simulink model "Aenea_model"  (R2020b)
settings: Solver=FixedStepDiscrete  StartTime=0.0  StopTime=10.0  FixedStep=0.02  RelTol=1e-3
values from neighbouring files (symbols this model uses):
  attuatore_Amax = deg2rad(27)    [AVVIO_AENEA_DATA.m]
  attuatore_Amin = deg2rad(-23)    [AVVIO_AENEA_DATA.m]
  attuatore_Emax = deg2rad(18)    [AVVIO_AENEA_DATA.m]
  attuatore_Emin = deg2rad(-32)    [AVVIO_AENEA_DATA.m]
  attuatore_Rmax = deg2rad(30)    [AVVIO_AENEA_DATA.m]
  attuatore_Rmin = deg2rad(-30)    [AVVIO_AENEA_DATA.m]
  attuatore_Tmax = 1    [AVVIO_AENEA_DATA.m]
  attuatore_Tmin = 0    [AVVIO_AENEA_DATA.m]
  interventoA_05 = 25    [AVVIO_AENEA_DATA.m]
  interventoA_1 = 20    [AVVIO_AENEA_DATA.m]
  interventoE_05 = 20    [AVVIO_AENEA_DATA.m]
  interventoE_1 = 15    [AVVIO_AENEA_DATA.m]
  interventoT = 0.1    [AVVIO_AENEA_DATA.m]
  inv_A = -1    [AVVIO_AENEA_DATA.m]
  inv_comp_h = -1    [AVVIO_AENEA_DATA.m]
  inv_E = 1    [AVVIO_AENEA_DATA.m]
  inv_R = 1    [AVVIO_AENEA_DATA.m]
  inv_T = 1    [AVVIO_AENEA_DATA.m]
  K_AW_B_AP_quota = 1000    [AVVIO_AENEA_DATA.m]
  K_AW_B_becc = -250    [AVVIO_AENEA_DATA.m]
  K_AW_B_imb = 0    [AVVIO_AENEA_DATA.m]
  K_AW_B_roll = 500    [AVVIO_AENEA_DATA.m]
  K_imb_inv = -1    [AVVIO_AENEA_DATA.m]
  Kd_h_app = 0.085    [AVVIO_AENEA_DATA.m]
  Kd_h_flare = 0.01    [AVVIO_AENEA_DATA.m]
  Ki_AP_quota_select = 0.014    [AVVIO_AENEA_DATA.m]
  Ki_AP_rotta = 0.03    [AVVIO_AENEA_DATA.m]
  Ki_AP_vel = 0.001*8    (= 0.008)    [AVVIO_AENEA_DATA.m]
  Ki_becch = -0.064065*10    (= -0.64065)    [AVVIO_AENEA_DATA.m]
  Ki_h_app = 0.055    [AVVIO_AENEA_DATA.m]
  Ki_h_cruise = 0.008    [AVVIO_AENEA_DATA.m]
  Ki_h_flare = 0.07    [AVVIO_AENEA_DATA.m]
  Ki_roll = 0.025*10    (= 0.25)    [AVVIO_AENEA_DATA.m]
  Kp_AP_quota_hold_h = 0.15    [AVVIO_AENEA_DATA.m]
  Kp_AP_quota_hold_l = 1    [AVVIO_AENEA_DATA.m]
  Kp_AP_quota_select = 0.014    [AVVIO_AENEA_DATA.m]
  Kp_AP_rotta = 0.7    [AVVIO_AENEA_DATA.m]
  Kp_AP_vel = 0.2692/8    (= 0.03365)    [AVVIO_AENEA_DATA.m]
  Kp_becch = -0.1918*10    (= -1.918)    [AVVIO_AENEA_DATA.m]
  Kp_comp_h = 0.035*15    (= 0.525)    [AVVIO_AENEA_DATA.m]
  Kp_h_app_max = 0.086    [AVVIO_AENEA_DATA.m]
  Kp_h_app_min = 0.01    [AVVIO_AENEA_DATA.m]
  Kp_h_cruise = 0.04    [AVVIO_AENEA_DATA.m]
  Kp_h_flare = 0.1    [AVVIO_AENEA_DATA.m]
  Kp_imb = -0.04*10    (= -0.4)    [AVVIO_AENEA_DATA.m]
  Kp_p = 0.025*5    (= 0.125)    [AVVIO_AENEA_DATA.m]
  Kp_q = -0.025*5    (= -0.125)    [AVVIO_AENEA_DATA.m]
  Kp_roll = 0.11*10    (= 1.1)    [AVVIO_AENEA_DATA.m]
  Kp_Rotta_ATO = 4    [AVVIO_AENEA_DATA.m]
  phi_max = deg2rad(30)    [AVVIO_AENEA_DATA.m]
  phi_min = deg2rad(-30)    [AVVIO_AENEA_DATA.m]
  pwm_aileron_max = 1940    [AVVIO_AENEA_DATA.m]
  pwm_aileron_min = 1099    [AVVIO_AENEA_DATA.m]
  pwm_elevator_max = 1939    [AVVIO_AENEA_DATA.m]
  pwm_elevator_min = 1099    [AVVIO_AENEA_DATA.m]
  pwm_rudder_max = 1971    [AVVIO_AENEA_DATA.m]
  pwm_rudder_min = 1130    [AVVIO_AENEA_DATA.m]
  pwm_throttle_max = 1940    [AVVIO_AENEA_DATA.m]
  pwm_throttle_min = 1160    [AVVIO_AENEA_DATA.m]
  safe_phi = 55    [AVVIO_AENEA_DATA.m]
  safe_V = 40    [AVVIO_AENEA_DATA.m]
  t_AP = 0.02    [AVVIO_AENEA_DATA.m]
  theta_max = deg2rad(15)    [AVVIO_AENEA_DATA.m]
  theta_min = deg2rad(-15)    [AVVIO_AENEA_DATA.m]
  time_alarm_SAFE = 1    [AVVIO_AENEA_DATA.m]
  V_max = 30    [AVVIO_AENEA_DATA.m]
  V_stall = 11    [AVVIO_AENEA_DATA.m]
  vel_wp1_al = 25    [AVVIO_AENEA_DATA.m]
  vel_wp2_al = 20    [AVVIO_AENEA_DATA.m]
undefined symbols (not defined in the file or in its folder): bias, DiscIntNeverNeededParam, Newton, Q1B, R1B, Raphson, Sensor_Offsets, tsamp, UP, vd_ini
libraries: simulink_extras x41, slpidlib x8, simulink x6, dspsigops x4, arduinolib x3, svdutilitieslib x3, aerolibtransform2sys x2, aerolibtransform2 x2, aerosimlib x2, cstblocks x1
(part 7 of 8)

== matlab function Aenea_model/AUTOPILOT_MODEL/AIR RX/MATLAB Function4 ==
  data: byte_pack input; status output; messaggio output; messaggio_2 output; byte_available input
function [status,messaggio,messaggio_2]  = Creazione_mavlink_message_2(byte_pack,byte_available)


persistent Interr_parz  message counter len_found mess_len

if isempty(Interr_parz)
    Interr_parz = false ;
end
if isempty(message)
     message = uint8(zeros(1,100 )) ;
end
if isempty (counter) 
    counter = uint8(0) ;    % variabile che conta quanti byte mancano per completare il messaggio
end 

if isempty(len_found) 
     len_found = false ;
end 

if isempty(mess_len) 
     mess_len = 0 ;
end 

status = 0;
M = length(byte_pack) ;
caso = 0 ;
messaggio = uint8(zeros(1,100 )) ;
messaggio_2 = uint8(zeros(1,100 )) ;
% LA VARIABILE INTERR_PARZ va attivata a 1 alla fine della funzone di
% lettura per indicare di leggere il successivo messaggio in arrivo 

[poss_254,num_254] = find_254(byte_pack) ;

if ((Interr_parz == true) && (num_254 == 1))                  % in questo caso verifico che il 254 sia effettivamente un altro inizio
if (poss_254(1) ~= counter+1)
   num_254 = 0; 
end
    
end



if ( num_254 == 1 && Interr_parz == false )             
    caso = 1 ;                                                            % 1 Messaggio Intero   o parziale che inizia                % attivare alla fine della funzione Interr_parz == true o false 
elseif (num_254 == 0 && Interr_parz == true )
    caso = 2 ;                                                        % 1 Messaggio Parziale senza inizio e poi nulla 
elseif (num_254 == 1 && Interr_parz == true )                         
    caso = 3 ;                                                        % 1 Messaggio Parziale e poi un altro messaggio completo o parziale
elseif  ( num_254 == 2 && Interr_parz == false ) 
    caso = 4 ;                                                         % Due messaggi completi  oppure 1 Completo + parziale ( attivare Interr_parz alla fine del codice)
end


switch (caso)
   
    
    
    case 1 
        pos_254 = poss_254(num_254) ;
        
        if pos_254 == M                                                                          % se il 254 sta alla fine 
             message(1) = byte_pack(pos_254)  ;
            len_found = false ;
            Interr_parz = true ;
        else
             len = byte_pack(pos_254 + 1)  ;
             if len <= 100
             if  ((byte_pack(poss_254(1)+1) + 8) == byte_available)                                             % se abbiamo tutto il messaggio all'interno del byte_pack
                message(1: 8 + len ) = byte_pack(pos_254 : pos_254 + (7+len) ) ;          % era cosi byte_pack(pos_254 : pos_254 + (8+len) ) ;
                messaggio = message ;
                status = 1 ;
                message = uint8(zeros(1,100 )) ;
                counter = uint8(0) ;
                len_found = true ;
                mess_len = 0 ;
             elseif ((byte_pack(poss_254(1)+1) + 8) > byte_available)
                mess_len = double(byte_available) ;                                       % lunghezza del messaggio da leggere dal byte_pack ( non uguale alla lunghezza del messaggio complessivo)
                message(1 : mess_len) = byte_pack(pos_254 : mess_len ) ;
                len_found = true ;
                counter = 8 + len - mess_len ;
                Interr_parz = true ;
             end
             else
                 messaggio = uint8(zeros(1,100 )) ;              
                 Interr_parz = false;
                 message = uint8(zeros(1,100 )) ;
                 counter = uint8(0) ;
                 len_found = false ;
                 mess_len = 0 ; 
                 status = 1 ;
             end   
             
        end
        
        
        
        
    case 2 
        
                                     % se la lunghezza è stata trovata e quindi ho il valore di counter che indica quante componenti mancano
           if byte_pack ~= 0
                message(mess_len + 1 : mess_len + counter) = byte_pack( 1 : counter) ;
                Interr_parz = false ;
                messaggio = message ;
                status = 1 ;
                message = uint8(zeros(1,100 )) ;
                len_found = true ;
                mess_len = 0 ;
                counter = uint8(0) ;
                
           else                                                    % se ho un messaggio parziale e nello step successivo non ricevo nulla allora azzero tutto, altrimenti entro in un loop infinito di messaggi sbagliati
                Interr_parz = false ;
                messaggio = uint8(zeros(1,100)) ;
                status = 1 ;
                message = uint8(zeros(1,100 )) ;
                len_found = true ;
                mess_len = 0 ;
                counter = uint8(0) ;  
           end        
        
        

  
        
    case 3 
        
                                     % se la lunghezza è stata trovata e quindi ho il valore di counter che indica quante componenti mancano
        pos_254 = poss_254(num_254) ;
        
                message(mess_len + 1 : mess_len + counter) = byte_pack( 1 : counter) ;
                Interr_parz = false ;
                messaggio = message ;
                status = 1 ;
                message = uint8(zeros(1,100 )) ;
                len_found = true ;
                mess_len = 0 ;
                counter = uint8(0) ;
                
             len = byte_pack(pos_254 + 1)  ;
             if len <= 100
             if  ((byte_pack(poss_254(1)+1) + 8) == uint8(byte_available-double(counter)))                                             % se abbiamo tutto il messaggio all'interno del byte_pack
                message(1: 8 + len ) = byte_pack(pos_254 : pos_254 + (7+len) ) ;          % era cosi byte_pack(pos_254 : pos_254 + (8+len) ) ;
                messaggio_2 = message ;
                status = 1 ;
                message = uint8(zeros(1,100 )) ;
                counter = uint8(0) ;
                len_found = true ;
                mess_len = 0 ;
             elseif ((byte_pack(poss_254(1)+1) + 8) > (uint8(byte_available)-counter))
                mess_len = double(byte_available) - double(counter) ;                                       % lunghezza del messaggio da leggere dal byte_pack ( non uguale alla lunghezza del messaggio complessivo)
                message(1 : mess_len) = byte_pack(pos_254 : mess_len ) ;
                len_found = true ;
                counter = 8 + len - mess_len ;
                Interr_parz = true ;
             end
             else
                 messaggio = uint8(zeros(1,100 )) ;              
                 Interr_parz = false;
                 message = uint8(zeros(1,100 )) ;
                 counter = uint8(0) ;
                 len_found = false ;
                 mess_len = 0 ; 
                 status = 1 ;
             end
                
      
            
        
        
        
      
        
        
    case 4
        primo_254 = poss_254(1) ;
        secondo_254 = poss_254(2) ;
        len_primo = byte_pack(primo_254 + 1) ;
    %    messaggio(1 : len_primo + 8) = byte_pack(primo_254 : primo_254 + (len_primo + 7)) ;           %era cosi      byte_pack(primo_254 : secondo_254 - 1)  ;

        if len_primo <= 100
        messaggio(1 : len_primo + 8) = byte_pack(primo_254 : primo_254 + (len_primo + 7)) ;             %era cosi      byte_pack(primo_254 : secondo_254 - 1)  ;
        else
        messaggio = uint8(zeros(1,100 )) ;
        Interr_parz = false;
        message = uint8(zeros(1,100 )) ;
        counter = uint8(0) ;
        len_found = false ;
        mess_len = 0 ;
        end
        
        status = 1;
        
             len = byte_pack(secondo_254 + 1)  ;
             if (len <= 100 && (secondo_254-primo_254 > 3))
             if ( (byte_available - ( secondo_254))  == 7 + len    )                                         % se abbiamo tutto il messaggio all'interno del byte_pack
                message(1: 8 + len ) = byte_pack(secondo_254 : secondo_254 + (7+len) ) ;      % era cosi byte_pack(pos_254 : pos_254 + (8+len) ) ;
                messaggio_2 = message ;
                status = 2 ;
                message = uint8(zeros(1,100 )) ;
                counter = uint8(0) ;
                len_found = true ;
                mess_len = 0 ;
             else
                mess_len = length(byte_pack(secondo_254:byte_available ) ) ;    % lunghezza del messaggio da leggere dal byte_pack ( non uguale alla lunghezza del messaggio complessivo)
                message(1 : mess_len) = byte_pack(secondo_254:byte_available ) ;
                len_found = true ;
                counter = 8 + len - mess_len ;
                Interr_parz = true ;
             end
             else
               messaggio_2 = uint8(zeros(1,100 )) ;              
               Interr_parz = false;
               message = uint8(zeros(1,100 )) ;
               counter = uint8(0) ;
               len_found = false ;
               mess_len = 0 ;    
              end
             
        
        
end
end






function [position,counter] = find_254(pack) 
    position = zeros(1,3) ;
    
    M = length(pack)  ;   
    counter = 0 ;
    for i = 1 : M
        if pack(i) == 254 
            counter = counter + 1;  
            position(counter) = i; 
        end
    end
    l = pack(position(1)+1);
    if counter > 1
    if ((pack(l+8+position(1)) ~= 254) && (position(1) ~= 0))
        counter = 1;
        position(2) = 0;
    end
    end
end

== stateflow chart Aenea_model/AUTOPILOT_MODEL/AUTOPILOTA/Subsystem1/Chart ==
  state AutoTakeoff
    Wp_selector = 0;
    Vec_selector = 0;
    Ato_selector = 1;
    Al_selector = 0;
    Go_home_selector = 0;
  state Waypoint
    Wp_selector = 1;
    Vec_selector = 0;
    Ato_selector = 0;
    Al_selector = 0;
    Go_home_selector = 0;
  state In
    Wp_selector = 0;
    Vec_selector = 0;
    Ato_selector = 0;
    Al_selector = 0;
    Go_home_selector = 0;
  state AutoLanding
    Wp_selector = 0;
    Vec_selector = 0;
    Ato_selector = 0;
    Al_selector = 1;
    Go_home_selector = 0;
  state Vettoriale
    Wp_selector = 0;
    Vec_selector = 1;
    Ato_selector = 0;
    Al_selector = 0;
    Go_home_selector = 0;
  state GoHome
    Wp_selector = 0;
    Vec_selector = 0;
    Ato_selector = 0;
    Al_selector = 0;
    Go_home_selector = 1;
  AutoTakeoff -> Waypoint [order 2] : [Ap_sel == 1 && modo == 1]
  Waypoint -> In [order 2] : [Ap_sel == 0]
  AutoTakeoff -> In [order 1] : [Ap_sel == 0]
  (default) -> In : {Wp_selector = 0;
      | Vec_selector = 0;
      | Ato_selector = 0;
      | Al_selector = 0;}
  Waypoint -> AutoLanding [order 4] : [Ap_sel == 1 && modo == 4]
  In -> Waypoint [order 1] : [Ap_sel == 1 && modo == 1]
  In -> AutoTakeoff [order 5] : [Ap_sel == 1 && modo == 3]
  AutoLanding -> Waypoint [order 3] : [Ap_sel == 1 && modo == 1]
  AutoLanding -> In [order 1] : [Ap_sel == 0]
  Vettoriale -> In [order 1] : [Ap_sel == 0]
  AutoTakeoff -> Vettoriale [order 3] : [Ap_sel == 1 && modo == 2]
  Waypoint -> GoHome [order 1] : [Ap_sel == 1&& modo == 5]
  Waypoint -> Vettoriale [order 3] : [Ap_sel == 1 && modo == 2]
  Vettoriale -> Waypoint [order 2] : [Ap_sel == 1 && modo == 1]
  In -> AutoLanding [order 4] : [Ap_sel == 1 && modo == 4]
  In -> GoHome [order 3] : [Ap_sel == 1 && modo == 5]
  GoHome -> In : [Ap_sel == 0]
  In -> Vettoriale [order 2] : [Ap_sel == 1 && modo == 2]
  Vettoriale -> AutoLanding [order 4] : [Ap_sel == 1 && modo == 4]
  AutoLanding -> Vettoriale [order 2] : [Ap_sel == 1 && modo == 2]
  AutoLanding -> GoHome [order 4] : [Ap_sel == 1 && modo == 5]
  Vettoriale -> GoHome [order 3] : [Ap_sel == 1&& modo == 5]
  data: Al_selector output; Ato_selector output; Go_home_selector output; Vec_selector output; Wp_selector output; modo input; Ap_sel input

== stateflow chart Aenea_model/AUTOPILOT_MODEL/AIR TX/Enable /Chart ==
  state sendbyte(bt,n) [function]
  state Inputblock
    entry: i=1;
    Inputblock -> (junction 28)
    (junction 32) -> (junction 28) [order 1] : [ i<Len]
        | {i++;}
    (junction 28) -> (junction 32) : {sendbyte(datain,i);}
    (junction 32) -> (junction 48) [order 2] : {i=1;}
  (default) -> Inputblock
  data: bt function_input uint8; n function_input; datain input uint8; Len input uint16 size=1; i local uint8 =0

== stateflow chart Aenea_model/AUTOPILOT_MODEL/AUTOPILOTA/AUTOPILOTI1/CONTROLLORE DI QUOTA/SELEZIONE MODALITA' HOLD//SELECT ==
  state Select
    during:
    mod=1;
  state Hold
    during:
    mod=0;
  (default) -> Select
  Select -> Hold : [deltah<10]
  Hold -> Select : [deltah>10]
  data: mod output double; deltah input

== matlab function Aenea_model/AUTOPILOT_MODEL/AIR TX/Heartbeat/Alarm set ==
  data: Alarm input; H_mav output; Rx_mode input

%%

function H_mav = Allarm_set(Alarm, Rx_mode)
%#cambia lo stato se c'è un allarme attivo
% Allarm: possibili allarmi proveniente dall'autopilota
% Rx_mode: richiesta da parte della stazione di terra
% H_mav: setto i parametri Base_mode e System_status del Heartbeat


H_mav = uint8(Rx_mode); % setta la modalità con quella ricevuta da terra

% se un allarme si attiva ha la precedenza sulla richiesta della QGC

if Alarm(1) == 1 % ovvero l'aereo è entrato in safe e si pone su traettoria circolare di sicurezza
    
    H_mav(1) = uint8(220); % MAV_MODE_AUTO_ARMED
    H_mav(2) = uint8(5);   % MAV_STATE_CRITICAL
%     H_mav(3) = uint8(128); % MAV_MODE_FLAG_SAFETY_ARMED

end

% se l'allareme di intervento pilota è attivo ha precedenza sull'allarm
% sefe per cui bisogna riscrivere lo stato del pilota

if Alarm(2) == 1 % si è attivato l'allarme dell'intervento pilota 
    
    H_mav(1) = uint8(216); % MAV_MODE_GUIDED_ARMED
    H_mav(2) = uint8(4);   % MAV_STATE_ACTIVE
%     H_mav(3) = uint8(8);   % MAV_MODE_FLAG_GUIDED_ENABLED

end

== matlab function Aenea_model/AUTOPILOT_MODEL/AIR TX/If_subsystem/iflogic_function ==
  data: H50 input; iflogic output; H10 input
function iflogic = fcn(H50,H10)
%#codegen
% prende in ingeresso i counter che contano il tempo
% e dice quale messaggio bisogna inviare in base alle frequenze scelte in
% Heartbeat:            1Hz
% SCALED_IMU:           20Hz
%attitude:              20Hz
%GLOBAL_POSITION_INT:   1Hz
%SYS_STATUS:            3Hz
%VFR_HUD:               2Hz
%SERVO_OUTPUT_RAW       1Hz
%SCALED_PRESSURE        1Hz

if H50 == 1  || H50==3
    iflogic=uint8(26); % SCALED_IMU 20Hz
elseif H50==2 || H50==4
    iflogic=uint8(30); %attitude 20Hz
elseif  H50==0 && H10==2
    iflogic=uint8(33); %GLOBAL_POSITION_INT 1Hz
elseif  H50==0 && H10==6
    iflogic=uint8(34); %GLOBAL_POSITION_INT_RAW 1Hz
elseif  H50==0 && H10==0
    iflogic=uint8(0); %Heartbeat 1Hz
elseif H50==0 && (H10==1 || H10==5 || H10==9)
    iflogic=uint8(1); %SYS_STATUS 3Hz
elseif H50==0 && (H10==3 || H10==8)
    iflogic=uint8(74); %VFR_HUD 2Hz
elseif H50==0 && (H10==7)
    iflogic=uint8(36); %SERVO_OUTPUT_RAW 1Hz
elseif H50==0 && (H10==4)
    iflogic=uint8(29); %SCALED_PRESSURE 1Hz
else
    iflogic=uint8(255); %non esiste nessun messaggio con questo codice
    
end

== stateflow chart Aenea_model/AUTOPILOT_MODEL/AUTOPILOTA/GESTIONE AUTOPILOTI1/ STATI ==
  state Go_Home
    during:
    modo = 5;
    switch_manetta = 1;
    switch_equilibratore =1;
    switch_alettoni=1;
    switch_timone=1;
  state MANUALE
    during:
    switch_manetta=0;
    switch_equilibratore=0;
    switch_alettoni=0;
    switch_timone=0;
  state Safe
    during:
    switch_manetta=1;
    switch_equilibratore=1;
    switch_alettoni=1;
    switch_timone=1;
    phi_safe=0.1745;
    theta_safe=0.05;
    throttle_safe=0.1;
  state Intervento_Pilota
    during:
    switch_manetta=0;
    switch_equilibratore=0;
    switch_alettoni=0;
    switch_timone=0;
  state AUTOMATICA
    state WAYPOINT
      during:
      modo = 1;
      switch_manetta = 1;
      switch_equilibratore =1;
      switch_alettoni=1;
      switch_timone=1;
    state TEST
      during:
      switch_manetta = 0;
      switch_equilibratore = 0;
      switch_alettoni = 0;
      switch_timone = 0;
    state VETTORIALE
      during:
      modo = 2;
      switch_manetta = 1;
      switch_equilibratore =1;
      switch_alettoni=1;
      switch_timone=1;
    state DECOLLO_AUTOMATICO
      during:
      modo = 3;
      switch_manetta = 1;
      switch_equilibratore = 1;
      switch_alettoni = 1;
      switch_timone = 1;
    state ATTERRAGGIO_AUTOMATICO
      during:
      modo = 4;
      switch_manetta = 1;
      switch_equilibratore =1;
      switch_alettoni=1;
      switch_timone=1;
    DECOLLO_AUTOMATICO -> WAYPOINT [order 2] : [WP_nav == 1 && h>30]
    TEST -> VETTORIALE : [test==0]
    WAYPOINT -> VETTORIALE [order 1] : [WP_nav == 0 &&  (IAS == 1 || ALT == 1 || HDG == 1||ATO==1)]
    (default) -> VETTORIALE
    VETTORIALE -> TEST [order 1] : [test==1]
    ATTERRAGGIO_AUTOMATICO -> WAYPOINT [order 1] : [AL==0 && h>20 && WP_nav==1 ]
    WAYPOINT -> ATTERRAGGIO_AUTOMATICO [order 2] : [AL==1]
    VETTORIALE -> WAYPOINT [order 4] : [WP_nav == 1]
    ATTERRAGGIO_AUTOMATICO -> VETTORIALE [order 2] : [AL==0 && h>20]
    DECOLLO_AUTOMATICO -> VETTORIALE [order 1] : [ATO == 0 && Tas >= 1 && (IAS == 1 || ALT == 1 || HDG == 1) ]
    VETTORIALE -> ATTERRAGGIO_AUTOMATICO [order 3] : [AL==1]
    VETTORIALE -> DECOLLO_AUTOMATICO [order 2] : [ATO == 1 && v_< 1]
    ATTERRAGGIO_AUTOMATICO -> DECOLLO_AUTOMATICO [order 3] : [ATO == 1 && AL == 0 && h<1 && v_<1]
  state Stand_By
    during:
    switch_manetta=0;
    switch_equilibratore=0;
    switch_alettoni=0;
    switch_timone=0;
  MANUALE -> Go_Home [order 1] : [Go_Home == 1 && Alarm_Safe == 0]
  Go_Home -> Intervento_Pilota [order 3] : [Alarm_Intervento==1]
  Go_Home -> Safe [order 2] : [Alarm_Safe == 1]
  (default) -> MANUALE
  AUTOMATICA -> Go_Home [order 3] : [Go_Home == 1]
  Go_Home -> AUTOMATICA [order 1] : [Go_Home == 0 && (WP_nav == 1 || IAS == 1 || ALT == 1 || HDG == 1|| AL == 1)]
  Safe -> MANUALE [order 2] : [MANUALE==1]
  Safe -> Intervento_Pilota [order 1] : [Alarm_Intervento==1]
  AUTOMATICA -> Safe [order 2] : [Alarm_Safe==1]
  Intervento_Pilota -> MANUALE : [MANUALE==1]
  AUTOMATICA -> Intervento_Pilota [order 1] : [Alarm_Intervento==1]
  AUTOMATICA -> MANUALE [order 5] : [MANUALE==1]
  Stand_By -> MANUALE [order 2] : [MANUALE==1]
  MANUALE -> Stand_By [order 2] : [MANUALE==0]
  Stand_By -> AUTOMATICA [order 1] : [Ingaggio_A_P==1]
  AUTOMATICA -> Stand_By [order 4] : [Ingaggio_A_P==0]
  data: MANUALE input; Ingaggio_A_P input; WP_nav input; ALT input; IAS input; HDG input; switch_manetta output double; switch_equilibratore output double; switch_alettoni output double; switch_timone output double; Alarm_Safe input; phi_safe output double; theta_safe output double; throttle_safe output double; Alarm_Intervento input; modo output double =1; ATO input; Tas input; AL input; v_ input; test input; h input; Go_Home input

== matlab function Aenea_model/AUTOPILOT_MODEL/AUTOPILOTA/GESTIONE AUTOPILOTI1/Intervento Manager/MATLAB Function1 ==
  data: Manuale input; Int_1 output; sw output; Ingaggio_AP input; absE input; absT input; interventoE_1 input; interventoE_05 input; Int_05 output; interventoT input
function [Int_1, sw, Int_05] = Intervento(Manuale, Ingaggio_AP, absE, absT, interventoE_1, interventoE_05, interventoT)
%#codegen

% persistent Ef Af Tf;
%
% if (isempty(Ef) || Manuale == 1 || Ingaggio_AP == 0)
%
%     Ef = absE;
%     Af = absA;
%     Tf = absT;
%
% end

persistent Tf;

if (isempty(Tf) || Manuale == 1 || Ingaggio_AP == 0)
    
    Tf = absT;
    
end

if Ingaggio_AP == 1
    
    %     dE = abs((Ef-absE));
    %     dA = abs((Af-absA));
    dT = abs((Tf-absT));
    
    %     if ((dE > 0.017 && dE < 0.1) && ALT == 1) % range compreso tra 0.97 e 5.73 deg di equilibratore
    
    if (absE > interventoE_1 && absE < interventoE_05) % interventoE_1 pari a 3.2 deg (il valore di trim dell'equilibratore alla massima velocità è di 3.18 deg)
        % interventoE_05 pari al 30% (7.5 deg) del valore massimo assumibile dall'equilibratore pari a 25 deg.
        % vedere il file Soglie_intervento.mat
        
        Int_1  = 1; % in questo caso scatta Int_temporiz il che significa che per attivarsi...
        Int_05 = 0; % l'intervento pilota deve essere soddisfatta anche la successiva...
        sw            = 1; % condizione sul tempo di durata del comando sull'equilibratore
        
        %     elseif (dE > 0.1 && ALT == 1)
        
    elseif absE > interventoE_05
        
        Int_1  = 0;
        Int_05 = 1;
        sw            = 0;
        
        %     elseif ((dA > 0.017 && dA < 0.087) && HDG == 1) % range compreso tra 0.97 e 4.98 deg di alettoni
        
    elseif dT > interventoT % interventoT uguale al 10% del valore massimo di manetta pari a 1; 0.1 sono circa tre scatti di comando della manetta
        
        Int_1  = 0; % nel caso della manetta se si supera la soglia scatta direttamente l'intervento pilota...
        Int_05 = 1; % senza il controllo sul tempo
        sw            = 0;
        
    else
        
        Int_1  = 0;
        Int_05 = 0;
        sw            = 1;
        
    end
    
else
    
    Int_1  = 0; % quando il velivolo è in modo manuale gli interruttori sono posti a zero
    Int_05 = 0;
    sw            = 1;
    
end

end

== matlab function Aenea_model/AUTOPILOT_MODEL/AIR TX/Waypoints/MATLAB Function ==
  data: WP_info_in input; WP_param_in input; WP_info output; GC_info input; WP_param output
function [WP_info,WP_param] = fcn(WP_info_in,WP_param_in, GC_info)
%#codegen
WP_info=WP_info_in(1,:); %%per sicurezza
WP_param=WP_param_in(1,:); %%per sicurezza
[m,n]=size(WP_info_in);
if GC_info(1)==2
    if GC_info(2)>=0 && GC_info(2)<m %per poter inviare i MISSION_ITEM
        WP_info=WP_info_in(GC_info(2)+1,:);
        WP_param=WP_param_in(GC_info(2)+1,:);
    end
end
if GC_info(1)==3 && GC_info(2)>=0 && GC_info(2)<200 %per poter inviae i MISSION_REQUEST
    WP_info=WP_info_in(GC_info(2)+1,:);
end

== matlab function Aenea_model/AUTOPILOT_MODEL/AUTOPILOTA/GESTIONE AUTOPILOTI1/MATLAB Function ==
  data: modo input; Switch_ATO output; Switch_AL output
function [Switch_ATO,Switch_AL] = fcn(modo)

persistent ATO AL

if modo == 3
    ATO = 1;
    AL = 0;
elseif modo == 4 
    AL = 1;
    ATO = 0;
else
    ATO = 0;
    AL = 0;
end

Switch_ATO = ATO;
Switch_AL = AL;

== matlab function Aenea_model/AUTOPILOT_MODEL/AUTOPILOTA/GESTIONE AUTOPILOTI1/Safe Manager/MATLAB Function1 ==
  data: Veloc input; phi input; Alarm_safe output; ingaggio_AP input; safe_V input; safe_phi input; Manuale input
function Alarm_safe = fcn(Veloc, phi, ingaggio_AP, safe_V, safe_phi, Manuale)
%#codegen
persistent alarm;

if (isempty(alarm))
    
    alarm = 0;

end

if (ingaggio_AP == 1 && (Veloc > safe_V || abs(phi) > safe_phi)) % soglia sulla velocità impostata a 40 m/s e soglia sull'angolo di rollio impostata a 45 deg
    
    alarm = 1;  

elseif (Manuale == 1) % l'allarme si disattiva solo quando si entra in modalità Manuale
    
    alarm = 0;

end 

Alarm_safe = alarm;

end

== matlab function Aenea_model/AUTOPILOT_MODEL/AUTOPILOTA/Subsystem1/Subsystem1/ALLINEAMENTO ==
  data: modo input; lat input; long input; h input; psi input; WP_db_info input; WP_db_param input; e_h output; vel output; lat_comandato output; long_comandato output; distance output; QUOTA output; ROTTA output; counter input; counter_out output
function [e_h,vel,lat_comandato,long_comandato,distance,QUOTA,ROTTA,counter_out] = autoland(modo,lat,long,h,psi,WP_db_info,WP_db_param,counter)
%#codegen
%WP_db_info=(nWP_tot n_WP frame command current autocontinue)
%per Nav
%WP_db_param=(velocità, autocontinue, vuoto, vuoto, lat_comandato, long_comandato, h_comandato)

persistent flag 

if isempty (flag)
    flag = 0;
end

%Definizione posizione waypoints
lat_comandato = WP_db_param(counter,5);
long_comandato = WP_db_param(counter,6);
h_comandato = WP_db_param(counter,7);

e_h = h_comandato - h; %errore quota

%Calcolo distanza velivolo-waypoint inseguito
a = (sin(((lat_comandato-lat)*pi/180)/2))^2+cos(lat*pi/180)*cos(lat_comandato*pi/180)*(sin(((long_comandato-long)*pi/180)/2))^2;
c = 2*atan2(sqrt(a),sqrt(1-a));
distance = 6378137*c;               

%Calcolo distanza velivolo-waypoint precedente
if counter > 1
    psi_ref = atan2(sin((WP_db_param(counter,6)-WP_db_param(counter-1,6))*pi/180)*cos(WP_db_param(counter,5)*pi/180),cos(WP_db_param(counter-1,5)*pi/180)*sin(WP_db_param(counter,5)*pi/180)-sin(WP_db_param(counter-1,5)*pi/180)*cos(WP_db_param(counter,5)*pi/180)*cos((WP_db_param(counter,6)-WP_db_param(counter-1,6))*pi/180))*180/pi;     %psi di riferimento
    a_pre = (sin(((lat-WP_db_param(counter-1,5))*pi/180)/2))^2+cos(WP_db_param(counter-1,5)*pi/180)*cos(lat*pi/180)*(sin(((long-WP_db_param(counter-1,6))*pi/180)/2))^2;
    c_pre = 2*atan2(sqrt(a_pre),sqrt(1-a_pre));
    dist = 6378137*c_pre;                                                  %distanza velivolo-WP precedente
else
    psi_ref = atan2(sin((long_comandato-long)*pi/180)*cos(lat_comandato*pi/180),cos(lat*pi/180)*sin(lat_comandato*pi/180)-sin(lat*pi/180)*cos(lat_comandato*pi/180)*cos((long_comandato-long)*pi/180))*180/pi;
    dist = 0;
end

if psi_ref < 0
    psi_ref = 360 - abs(psi_ref);
end

autocontinue=WP_db_param(counter,2); 

%Definizione angolo tra WP successivi
if autocontinue == 1
    a_fut = (sin(((WP_db_param(counter+1,5)-WP_db_param(counter,5))*pi/180)/2))^2+cos(WP_db_param(counter,5)*pi/180)*cos(WP_db_param(counter+1,5)*pi/180)*(sin(((WP_db_param(counter+1,6)-WP_db_param(counter,6))*pi/180)/2))^2;
    c_fut = 2*atan2(sqrt(a_fut),sqrt(1-a_fut));
    dist_fut = 6378137*c_fut;    %distanza waypoint inseguito - waypoint successivo
    psi_ref_fut = atan2(sin((WP_db_param(counter+1,6)-WP_db_param(counter,6))*pi/180)*cos(WP_db_param(counter+1,5)*pi/180),cos(WP_db_param(counter,5)*pi/180)*sin(WP_db_param(counter+1,5)*pi/180)-sin(WP_db_param(counter,5)*pi/180)*cos(WP_db_param(counter+1,5)*pi/180)*cos((WP_db_param(counter+1,6)-WP_db_param(counter,6))*pi/180))*180/pi;      %distanza WP-WP+1
    if psi_ref_fut < 0
        psi_ref_fut = 360 - abs(psi_ref_fut);
    end
    if counter > 1
        angoloWP = abs(psi_ref_fut - psi_ref);
    else 
        angoloWP = abs(psi_ref_fut - (atan2(sin((long_comandato-long)*pi/180)*cos(lat_comandato*pi/180),cos(lat*pi/180)*sin(lat_comandato*pi/180)-sin(lat*pi/180)*cos(lat_comandato*pi/180)*cos((long_comandato-long)*pi/180))*180/pi));
    end
else
    dist_fut = 0;
    angoloWP = 0;
end


if counter < 2
    angoloWP_pre = 0;
elseif counter == 2
    angoloWP_pre = abs(psi_ref - atan2(sin((WP_db_param(counter-1,6)-long)*pi/180)*cos(WP_db_param(counter-1,5)*pi/180),cos(lat*pi/180)*sin(WP_db_param(counter-1,5)*pi/180)-sin(lat*pi/180)*cos(WP_db_param(counter-1,5)*pi/180)*cos((WP_db_param(counter-1,6)-long)*pi/180))*180/pi);
else
    psi_ref_pre = atan2(sin((WP_db_param(counter-1,6)-WP_db_param(counter-2,6))*pi/180)*cos(WP_db_param(counter-1,5)*pi/180),cos(WP_db_param(counter-2,5)*pi/180)*sin(WP_db_param(counter-1,5)*pi/180)-sin(WP_db_param(counter-2,5)*pi/180)*cos(WP_db_param(counter-1,5)*pi/180)*cos((WP_db_param(counter-1,6)-WP_db_param(counter-2,6))*pi/180))*180/pi;
if psi_ref_pre < 0
    psi_ref_pre = 360 - abs(psi_ref_pre);
end
    angoloWP_pre = abs(psi_ref - psi_ref_pre);
end
    
if angoloWP <=3                                  % Condizione aggiunta da Sensolini, altrimenti l'errore in atterraggio era troppo grande
    error = 1;
    tolleranza_distWP_fut = 20;
elseif angoloWP <= 10
    error = 30;                                       %Definizione raggio di errore 
    tolleranza_distWP_fut = 100;                      %Definizione distanza minima accettabile tra WP successivi
elseif angoloWP > 10 && angoloWP <= 50 
    error = 80;
    tolleranza_distWP_fut = 250;
elseif angoloWP > 50 && angoloWP <= 90     
    error = 100;
    tolleranza_distWP_fut = 300;
elseif angoloWP > 90 && angoloWP <= 120     
    error = 150;
    tolleranza_distWP_fut = 350;
else     
    error = 200;
    tolleranza_distWP_fut = 400;
end

nWP=size(WP_db_param,1);

%Definizione distanza dal WP precedente per correzione traiettoria

if angoloWP_pre <= 10
    soglia_dist = 80;                                   
elseif angoloWP_pre > 10 && angoloWP_pre <= 50 
    soglia_dist = 200;
elseif angoloWP_pre > 50 && angoloWP_pre <= 90 
    soglia_dist = 300;
elseif angoloWP_pre > 90 && angoloWP_pre <= 120 
    soglia_dist = 350;
else
    soglia_dist = 400;
end

k=1.3;    %fattore moltiplicativo correzione rotta

%Definizione rotta
if autocontinue == 1  
    
    psi_comandato = atan2(sin((long_comandato - long)*pi/180)*cos(lat_comandato*pi/180),cos(lat*pi/180)*sin(lat_comandato*pi/180)-sin(lat*pi/180)*cos(lat_comandato*pi/180)*cos((long_comandato - long)*pi/180))*180/pi;     %rotta da seguire
    vel = WP_db_param(counter,1);                   %velocità di approccio al wp
    psi_comandato_fut = atan2(sin((WP_db_param(counter+1,6)-long)*pi/180)*cos(WP_db_param(counter+1,5)*pi/180),cos(lat*pi/180)*sin(WP_db_param(counter+1,5)*pi/180)-sin(lat*pi/180)*cos(WP_db_param(counter+1,5)*pi/180)*cos((WP_db_param(counter+1,6)-long)*pi/180))*180/pi;
    
    if vel <= 20                                    %Definizione raggio di errore in base alla velocità di volo
        error = error*1.1;
    elseif (vel <= 25 && vel > 20)
        error = error*1.2;
    elseif (vel <= 30 && vel > 25)
        error = error*1.3;
    else 
        error = error*1.4;
    end
    
        if dist < soglia_dist && distance > error
            psi_comandato = atan2(sin((long_comandato - long)*pi/180)*cos(lat_comandato*pi/180),cos(lat*pi/180)*sin(lat_comandato*pi/180)-sin(lat*pi/180)*cos(lat_comandato*pi/180)*cos((long_comandato - long)*pi/180))*180/pi;
        elseif dist > soglia_dist && distance > error
            psi_comandato = atan2(sin((long_comandato - long)*pi/180)*cos(lat_comandato*pi/180),cos(lat*pi/180)*sin(lat_comandato*pi/180)-sin(lat*pi/180)*cos(lat_comandato*pi/180)*cos((long_comandato - long)*pi/180))*180/pi;
            err = abs ( psi_comandato - psi_ref );             %errore inseguimento rotta
            if (psi_ref <= 90 && psi_ref >= 0)                 %primo quadrante
                if psi_comandato > psi_ref
                    psi_comandato = psi_comandato + k*err;
                elseif psi_comandato < psi_ref
                    psi_comandato = psi_comandato - k*err;
                else
                    psi_comandato = psi_comandato;
                end                   
            elseif (psi_ref <= 180 && psi_ref > 90)             %quarto quadrante
                if psi_ref*psi_comandato > 0
                    if psi_comandato > psi_ref || ( psi_comandato < -90 && psi_comandato > -180)
                        psi_comandato = psi_comandato + k*err;
                    elseif psi_comandato < psi_ref
                        psi_comandato = psi_comandato - k*err;
                    else
                        psi_comandato = psi_comandato;
                    end                      
                else
                    err = abs ( 360 - abs(psi_comandato) - psi_ref); 
                    if psi_comandato > psi_ref || ( psi_comandato < -90 && psi_comandato > -180)
                        psi_comandato = psi_comandato + k*err;
                    elseif psi_comandato < psi_ref
                        psi_comandato = psi_comandato - k*err;
                    else
                        psi_comandato = psi_comandato;
                    end                     
                end
            elseif(psi_ref < -90 && psi_ref >= -180)             %terzo quadrante
                if psi_ref*psi_comandato > 0
                    if psi_comandato > psi_ref
                        psi_comandato = psi_comandato + k*err;
                    elseif psi_comandato < psi_ref  || (psi_comandato < 180 && psi_comandato > 90)
                        psi_comandato = psi_comandato - k*err;
                    else
                        psi_comandato = psi_comandato;
                    end  
                else
                    err = abs ( 360 -(psi_comandato) - abs(psi_ref)); 
                    if psi_comandato > psi_ref
                        psi_comandato = psi_comandato + k*err;
                    elseif psi_comandato < psi_ref || (psi_comandato < 180 && psi_comandato > 90)
                        psi_comandato = psi_comandato - k*err;
                    else
                        psi_comandato = psi_comandato;
                    end                     
                end
            elseif(psi_ref < 0 && psi_ref >= -90)             %secondo quadrante
                if psi_comandato > psi_ref
                    psi_comandato = psi_comandato + k*err;
                elseif psi_comandato < psi_ref
                    psi_comandato = psi_comandato - k*err;
                else
                    psi_comandato = psi_comandato;
                end
            end
            
        elseif distance < error
            if dist_fut > tolleranza_distWP_fut
                psi_comandato = psi_comandato_fut;
                counter = counter + 1;
            else
                if counter < nWP-1
                    counter = counter + 2;
                else
                    vel=22;
                    h_comandato=h+0.4;
                    psi_comandato=psi+36.6;   
                    e_h=0;
                    flag=1;
                end
            end
        end
         
    
else
    
    psi_comandato = atan2(sin((long_comandato - long)*pi/180)*cos(lat_comandato*pi/180),cos(lat*pi/180)*sin(lat_comandato*pi/180)-sin(lat*pi/180)*cos(lat_comandato*pi/180)*cos((long_comandato - long)*pi/180))*180/pi;
    vel = WP_db_param(counter,1);                   
    error = 40;
    
        if dist < soglia_dist && flag == 0
                  psi_comandato = atan2(sin((long_comandato - long)*pi/180)*cos(lat_comandato*pi/180),cos(lat*pi/180)*sin(lat_comandato*pi/180)-sin(lat*pi/180)*cos(lat_comandato*pi/180)*cos((long_comandato - long)*pi/180))*180/pi;
        elseif dist > soglia_dist && distance > error && flag == 0
                err = abs ( psi_comandato - psi_ref );        
                if (psi_ref <= 90 && psi_ref >= 0)                 %primo quadrante
                    if psi_comandato > psi_ref
                        psi_comandato = psi_comandato + k*err;
                    elseif psi_comandato < psi_ref
                        psi_comandato = psi_comandato - k*err;
                    else
                        psi_comandato = psi_comandato;
                    end 
                elseif (psi_ref <= 180 && psi_ref > 90)             %quarto quadrante
                    if psi_ref*psi_comandato > 0
                        if psi_comandato > psi_ref || ( psi_comandato < -90 && psi_comandato > -180)
                            psi_comandato = psi_comandato + k*err;
                        elseif psi_comandato < psi_ref
                            psi_comandato = psi_comandato - k*err;
                        else
                            psi_comandato = psi_comandato;
                        end
                    else
                        err = abs ( 360 - abs(psi_comandato) - psi_ref); 
                        if psi_comandato > psi_ref || ( psi_comandato < -90 && psi_comandato > -180)
                            psi_comandato = psi_comandato + k*err;
                        elseif psi_comandato < psi_ref
                            psi_comandato = psi_comandato - k*err;
                        else
                            psi_comandato = psi_comandato;
                        end                     
                    end
                elseif(psi_ref < -90 && psi_ref >= -180)             %terzo quadrante
                    if psi_ref*psi_comandato > 0
                        if psi_comandato > psi_ref
                            psi_comandato = psi_comandato + k*err;
                        elseif psi_comandato < psi_ref  || (psi_comandato < 180 && psi_comandato > 90)
                            psi_comandato = psi_comandato - k*err;
                        else
                            psi_comandato = psi_comandato;
                        end 
                    else
                        err = abs ( 360 -(psi_comandato) - abs(psi_ref)); 
                        if psi_comandato > psi_ref
                            psi_comandato = psi_comandato + k*err;
                        elseif psi_comandato < psi_ref || (psi_comandato < 180 && psi_comandato > 90)
                            psi_comandato = psi_comandato - k*err;
                        else
                            psi_comandato = psi_comandato;
                        end                         
                    end
                elseif(psi_ref < 0 && psi_ref >= -90)             %secondo quadrante
                    if psi_comandato > psi_ref
                        psi_comandato = psi_comandato + k*err;
                    elseif psi_comandato < psi_ref
                        psi_comandato = psi_comandato - k*err;
                    else
                        psi_comandato = psi_comandato;
                    end
                end
                
        else            
                vel=22;
                h_comandato=h+0.4;
                psi_comandato=psi+36.6;   
                e_h=0;
                flag=1;                       %con flag=1 l'aereo rimane in loiter senza uscire dal ciclo            
        end
          
end


%se ho nWPtotali=0 (lat,long,alt==0), traiettoria circolare
if lat_comandato == 0 && long_comandato == 0 && h_comandato==0    
    h_comandato=h+0.3;
    psi_comandato=psi+36.6;   
    vel=22;
    e_h=0;   
end

%output  
QUOTA = h_comandato;
ROTTA = psi_comandato;


%se arrivo all'ultimo WP, loiter 
if counter == size(WP_db_param,1) && autocontinue > 0    
    autocontinue = 0;     
end

%I waipoint si resettano una volta conclusa la manovra
if modo == 4
    counter_out = counter;
else
    counter_out = 1;    
end

== matlab function Aenea_model/AUTOPILOT_MODEL/AUTOPILOTA/Subsystem1/Subsystem1/FLARE/MATLAB Function ==
  data: WP_db_param input; rotta output; lat input; long input
function rotta  = rotta(WP_db_param,lat,long)
%#codegen

lat_comandato = WP_db_param(3,5);      
long_comandato = WP_db_param(3,6);


psi_ref = atan2(sin((WP_db_param(3,6)-WP_db_param(2,6))*pi/180)*cos(WP_db_param(3,5)*pi/180),cos(WP_db_param(2,5)*pi/180)*sin(WP_db_param(3,5)*pi/180)-sin(WP_db_param(2,5)*pi/180)*cos(WP_db_param(3,5)*pi/180)*cos((WP_db_param(3,6)-WP_db_param(2,6))*pi/180))*180/pi;     %psi di riferimento

psi_comandato = atan2(sin((long_comandato - long)*pi/180)*cos(lat_comandato*pi/180),cos(lat*pi/180)*sin(lat_comandato*pi/180)-sin(lat*pi/180)*cos(lat_comandato*pi/180)*cos((long_comandato - long)*pi/180))*180/pi;
err = abs ( psi_comandato - psi_ref ); 
k = 1.4;

if (psi_ref <= 90 && psi_ref >= 0)                 %primo quadrante
                    if psi_comandato > psi_ref
                        psi_comandato = psi_comandato + k*err;
                    elseif psi_comandato < psi_ref
                        psi_comandato = psi_comandato - k*err;
                    else
                        psi_comandato = psi_comandato;
                    end
elseif (psi_ref <= 180 && psi_ref > 90)             %quarto quadrante
                    if psi_ref*psi_comandato > 0
                        if psi_comandato > psi_ref || ( psi_comandato < -90 && psi_comandato > -180)
                            psi_comandato = psi_comandato + k*err;
                        elseif psi_comandato < psi_ref
                            psi_comandato = psi_comandato - k*err;
                        else
                            psi_comandato = psi_comandato;
                        end                      
                    else
                        err = abs ( 360 - abs(psi_comandato) - psi_ref); 
                        if psi_comandato > psi_ref || ( psi_comandato < -90 && psi_comandato > -180)
                            psi_comandato = psi_comandato + k*err;
                        elseif psi_comandato < psi_ref
                            psi_comandato = psi_comandato - k*err;
                        else
                            psi_comandato = psi_comandato;
                        end                     
                    end
elseif(psi_ref < -90 && psi_ref >= -180)             %terzo quadrante
                    if psi_ref*psi_comandato > 0
                        if psi_comandato > psi_ref
                            psi_comandato = psi_comandato + k*err;
                        elseif psi_comandato < psi_ref  || (psi_comandato < 180 && psi_comandato > 90)
                            psi_comandato = psi_comandato - k*err;
                        else
                            psi_comandato = psi_comandato;
                        end  
                    else
                        err = abs ( 360 -(psi_comandato) - abs(psi_ref)); 
                        if psi_comandato > psi_ref
                            psi_comandato = psi_comandato + k*err;
                        elseif psi_comandato < psi_ref || (psi_comandato < 180 && psi_comandato > 90)
                            psi_comandato = psi_comandato - k*err;
                        else
                            psi_comandato = psi_comandato;
                        end                     
                    end
elseif(psi_ref < 0 && psi_ref >= -90)             %secondo quadrante
                    if psi_comandato > psi_ref
                        psi_comandato = psi_comandato + k*err;
                    elseif psi_comandato < psi_ref
                        psi_comandato = psi_comandato - k*err;
                    else
                        psi_comandato = psi_comandato;
                    end
end

rotta = psi_comandato;

== matlab function Aenea_model/AUTOPILOT_MODEL/AIR RX/MATLAB Function2 ==
  data: mess_out output; Len output; status input; mess_1 input; mess_2 input; buff_prev input; buffer output
function [mess_out,Len,buffer] = fcn(status,mess_1,mess_2,buff_prev)


mess_out=uint8(zeros(1,100));
buffer = uint8(zeros(3,100));
counter = uint8(0);
Len = int32(0);



mess_out = buff_prev(3,:);       %il messaggio in uscita è l'ultima riga
Len = int32(mess_out(1,2));



buffer(1,:) = uint8(zeros(1,100)); %buffer è buff_prev traslato in basso di 1 riga, quindi elimino mess_out
for j=2:1:3
buffer(j,:) = buff_prev(j-1,:);
end
i=3;
while i >= 1                        %cerco la prima riga nulla dal basso
    if buffer(i,:) == 0
        counter = uint8(i);
        break
    end
    i = i-1;
end


if status == 1                   
    buffer(counter,:) = mess_1;
    
elseif status == 2
    buffer(counter,:) = mess_1;
    buffer(counter-1,:) = mess_2;
    
    
else
    buffer(counter,:) = uint8(zeros(1,100));


end



end

== matlab function Aenea_model/AUTOPILOT_MODEL/AUTOPILOTA/Subsystem1/Subsystem1/CREAZIONE_WAYPOINT /AUTOLANDING_WAYPOINTS ==
  data: WP_info output; WP_param output; Lat_Home input; Long_Home input; h_Home input; alt input; vel_wp1_al input; vel_wp2_al input

function [WP_info,WP_param]  = fcn(Lat_Home,Long_Home,h_Home,alt,vel_wp1_al,vel_wp2_al)
%#codegen

WP_info=zeros(3,6);
WP_param=zeros(3,7);


for i=1:3

    WP_info(i,1)=3;                 %
    WP_info(i,2)=i-1;               % numero del waypoint da 1 a 6
    WP_info(i,3)=16;                % commande del tipo del command
    WP_info(i,4)=0;                 % sistema di riferimento
    WP_info(i,5)=0;                 % current waypoint
    WP_info(i,6)=1;                 %
    
    
    
    
WP_param(i,1)=vel_wp2_al;               %Velocita del WP
WP_param(i,2)=1;                % Autocontinue 1
WP_param(i,3)=0;                % Parametro  non utilizzato
WP_param(i,4)=0;                % Parametro  non utilizzato
WP_param(i,5)=Lat_Home(i);      % LAT
WP_param(i,6)=Long_Home(i);     % LONG
WP_param(i,7)=h_Home+alt(i);    % ALT
    
    
end

WP_param(1,1)=vel_wp1_al;
WP_param(3,2)=0;                % Autocontinue 1

end

== matlab function Aenea_model/AUTOPILOT_MODEL/AUTOPILOTA/Subsystem1/Subsystem3/GO_HOME ==
  data: lat input; V_goHome output; long input; h input; psi input; Lat_Home input; Long_Home input; h_goHome_rif input; V_goHome_rif input; h_goHome output; RC_goHome output; rotta_goHome output
function [V_goHome, h_goHome, RC_goHome, rotta_goHome] = go_home(lat, long, h, psi, Lat_Home, Long_Home, h_goHome_rif, V_goHome_rif)

persistent flag
if isempty (flag)
    flag = 0;
end

lat_comandato = Lat_Home;
long_comandato = Long_Home;

a = (sin(((lat_comandato-lat)*pi/180)/2))^2+cos(lat*pi/180)*cos(lat_comandato*pi/180)*(sin(((long_comandato-long)*pi/180)/2))^2;
c = 2*atan2(sqrt(a),sqrt(1-a));
distance = 6378137*c; 

rotta_goHome = atan2(sin((long_comandato - long)*pi/180)*cos(lat_comandato*pi/180),cos(lat*pi/180)*sin(lat_comandato*pi/180)-sin(lat*pi/180)*cos(lat_comandato*pi/180)*cos((long_comandato - long)*pi/180))*180/pi;     %rotta da seguire
h_goHome = h_goHome_rif;
V_goHome = V_goHome_rif;
RC_goHome = h_goHome - h;

    if distance < 30 && flag == 0
        flag = 1;
        V_goHome = V_goHome_rif;
        h_goHome = h_goHome_rif + 0.4;
        rotta_goHome = psi + 100;
        RC_goHome = 0;
    end
end

== matlab function Aenea_model/AUTOPILOT_MODEL/AIR RX/MATLAB Function3 ==
  data: mess_out input; new_mex output; mess_out_prev input
function new_mex = fcn(mess_out,mess_out_prev)
persistent counter

if isempty(counter)
    counter = uint16(0);
end

new_mex = uint16(0);


if ( mess_out(3) ~= mess_out_prev(3) && (all(mess_out ~= 0) == false) )

    if counter > 100
        counter = uint16(0);
    end
    counter = counter +1;
end
new_mex = counter;

end
